simulink model "Relu_NoOutFB_4_4_1_HW_C6"  (R2012b)
settings: Solver=FixedStepDiscrete  SolverMode=SingleTasking  StartTime=0.0  StopTime=limSim  FixedStep=ts  RelTol=1e-3
undefined symbols (not defined in the file): alpha, delayMulx, delayMuly, delayROMSig, M2, M3, mu, ts
libraries: xbsIndex_r4 x1578, roblocks x1
(part 10 of 13)

== system Relu_NoOutFB_4_4_1_HW_C6/EN_MLP_BK_(1,4_NL,1_L)_HW_FPGA2/MLP_BK_(2,4_NL,1_L)_HW_FPGA/BK (2,4_NL,1_L)/Subsystem8/Subsystem2 ==
  Gx_1(n) : Inport
  x_1(n) : Inport  Port=2
  AddSub1 : xbsIndex_r4/AddSub  mode=Addition  use_carryin=off  use_carryout=off  en=off  latency=0  precision=User Defined  arith_type="Signed  (2's comp)"  n_bits=nb  bin_pt=bp  quantization=Truncate  overflow=Wrap  dbl_ovrd=off  use_behavioral_HDL=off  hw_selection=Fabric  pipelined=off  block_type=addsub
  AddSub2 : xbsIndex_r4/AddSub  mode=Addition  use_carryin=off  use_carryout=off  en=off  latency=0  precision=User Defined  arith_type="Signed  (2's comp)"  n_bits=nb  bin_pt=bp  quantization=Truncate  overflow=Wrap  dbl_ovrd=off  use_behavioral_HDL=off  hw_selection=Fabric  pipelined=off  block_type=addsub
  CMult : xbsIndex_r4/CMult  const=mu  gui_display_data_type=Fixed-point  const_n_bits=32  const_bin_pt=32  float_type=Single  exp_bits=8  fraction_bits=24  en=off  latency=0  precision=User Defined  arith_type="Signed  (2's comp)"  n_bits=nb  bin_pt=bp  quantization="Round  (unbiased: +/- Inf)"  overflow=Wrap  dbl_ovrd=off  use_behavioral_HDL=off  mem_type=Distributed RAM  pipeline=off  block_type=cmult
  CMult2 : xbsIndex_r4/CMult  const=alpha  gui_display_data_type=Fixed-point  const_n_bits=32  const_bin_pt=32  float_type=Single  exp_bits=8  fraction_bits=24  en=off  latency=0  precision=User Defined  arith_type="Signed  (2's comp)"  n_bits=nb  bin_pt=bp  quantization="Round  (unbiased: +/- Inf)"  overflow=Wrap  dbl_ovrd=off  use_behavioral_HDL=off  mem_type=Distributed RAM  pipeline=off  block_type=cmult
  Register : xbsIndex_r4/Register  init=real(M3(1,4))  rst=off  en=off  dbl_ovrd=off  block_type=register
  Register1 : xbsIndex_r4/Register  init=0  rst=off  en=off  dbl_ovrd=off  block_type=register
  w_ij(n)*Gy(n)2 : xbsIndex_r4/Mult  precision=User Defined  arith_type="Signed  (2's comp)"  n_bits=nb  bin_pt=bp  quantization="Round  (unbiased: +/- Inf)"  overflow=Saturate  en=off  latency=delayMulx  dbl_ovrd=off  use_behavioral_HDL=off  opt=Speed  use_embedded=on  optimum_pipeline=off  pipeline=on  use_rpm=on  placement_style=Triangular  block_type=mult
  Wx_13(n) : Outport
  wires:
  x_1(n)/1 -> w_ij(n)*Gy(n)2/2
  w_ij(n)*Gy(n)2/1 -> CMult/1
  CMult/1 -> AddSub2/2  "dw(n) = z_0(n)*e(n)*mu"
  AddSub2/1 -> AddSub1/2
  AddSub1/1 -> Register/1  "w_ij(n+1)"
  Register1/1 -> CMult2/1  "w_ij(n-1)"
  CMult2/1 -> AddSub2/1  "alpha*w_ij(n-1)"
  Register/1 -> AddSub1/1, Register1/1, Wx_13(n)/1  "w_ij(n)"
  Gx_1(n)/1 -> w_ij(n)*Gy(n)2/1

== system Relu_NoOutFB_4_4_1_HW_C6/EN_MLP_BK_(1,4_NL,1_L)_HW_FPGA2/MLP_BK_(2,4_NL,1_L)_HW_FPGA/BK (2,4_NL,1_L)/Subsystem8/Subsystem3 ==
  Gx_1(n) : Inport
  x_1(n) : Inport  Port=2
  AddSub1 : xbsIndex_r4/AddSub  mode=Addition  use_carryin=off  use_carryout=off  en=off  latency=0  precision=User Defined  arith_type="Signed  (2's comp)"  n_bits=nb  bin_pt=bp  quantization=Truncate  overflow=Wrap  dbl_ovrd=off  use_behavioral_HDL=off  hw_selection=Fabric  pipelined=off  block_type=addsub
  AddSub2 : xbsIndex_r4/AddSub  mode=Addition  use_carryin=off  use_carryout=off  en=off  latency=0  precision=User Defined  arith_type="Signed  (2's comp)"  n_bits=nb  bin_pt=bp  quantization=Truncate  overflow=Wrap  dbl_ovrd=off  use_behavioral_HDL=off  hw_selection=Fabric  pipelined=off  block_type=addsub
  CMult : xbsIndex_r4/CMult  const=mu  gui_display_data_type=Fixed-point  const_n_bits=32  const_bin_pt=32  float_type=Single  exp_bits=8  fraction_bits=24  en=off  latency=0  precision=User Defined  arith_type="Signed  (2's comp)"  n_bits=nb  bin_pt=bp  quantization="Round  (unbiased: +/- Inf)"  overflow=Wrap  dbl_ovrd=off  use_behavioral_HDL=off  mem_type=Distributed RAM  pipeline=off  block_type=cmult
  CMult2 : xbsIndex_r4/CMult  const=alpha  gui_display_data_type=Fixed-point  const_n_bits=32  const_bin_pt=32  float_type=Single  exp_bits=8  fraction_bits=24  en=off  latency=0  precision=User Defined  arith_type="Signed  (2's comp)"  n_bits=nb  bin_pt=bp  quantization="Round  (unbiased: +/- Inf)"  overflow=Wrap  dbl_ovrd=off  use_behavioral_HDL=off  mem_type=Distributed RAM  pipeline=off  block_type=cmult
  Register : xbsIndex_r4/Register  init=real(M3(1,5))  rst=off  en=off  dbl_ovrd=off  block_type=register
  Register1 : xbsIndex_r4/Register  init=0  rst=off  en=off  dbl_ovrd=off  block_type=register
  w_ij(n)*Gy(n)2 : xbsIndex_r4/Mult  precision=User Defined  arith_type="Signed  (2's comp)"  n_bits=nb  bin_pt=bp  quantization="Round  (unbiased: +/- Inf)"  overflow=Saturate  en=off  latency=delayMulx  dbl_ovrd=off  use_behavioral_HDL=off  opt=Speed  use_embedded=on  optimum_pipeline=off  pipeline=on  use_rpm=on  placement_style=Triangular  block_type=mult
  Wx_14(n) : Outport
  wires:
  Gx_1(n)/1 -> w_ij(n)*Gy(n)2/1
  Register/1 -> Wx_14(n)/1, Register1/1, AddSub1/1  "w_ij(n)"
  CMult2/1 -> AddSub2/1  "alpha*w_ij(n-1)"
  Register1/1 -> CMult2/1  "w_ij(n-1)"
  AddSub1/1 -> Register/1  "w_ij(n+1)"
  AddSub2/1 -> AddSub1/2
  CMult/1 -> AddSub2/2  "dw(n) = z_0(n)*e(n)*mu"
  w_ij(n)*Gy(n)2/1 -> CMult/1
  x_1(n)/1 -> w_ij(n)*Gy(n)2/2

== system Relu_NoOutFB_4_4_1_HW_C6/EN_MLP_BK_(1,4_NL,1_L)_HW_FPGA2/MLP_BK_(2,4_NL,1_L)_HW_FPGA/BK (2,4_NL,1_L)/Subsystem8/Subsystem5 ==
  Gx_1(n) : Inport
  x_0(n) : Inport  Port=2
  AddSub1 : xbsIndex_r4/AddSub  mode=Addition  use_carryin=off  use_carryout=off  en=off  latency=0  precision=User Defined  arith_type="Signed  (2's comp)"  n_bits=nb  bin_pt=bp  quantization=Truncate  overflow=Wrap  dbl_ovrd=off  use_behavioral_HDL=off  hw_selection=Fabric  pipelined=off  block_type=addsub
  AddSub2 : xbsIndex_r4/AddSub  mode=Addition  use_carryin=off  use_carryout=off  en=off  latency=0  precision=User Defined  arith_type="Signed  (2's comp)"  n_bits=nb  bin_pt=bp  quantization=Truncate  overflow=Wrap  dbl_ovrd=off  use_behavioral_HDL=off  hw_selection=Fabric  pipelined=off  block_type=addsub
  CMult : xbsIndex_r4/CMult  const=mu  gui_display_data_type=Fixed-point  const_n_bits=32  const_bin_pt=32  float_type=Single  exp_bits=8  fraction_bits=24  en=off  latency=0  precision=User Defined  arith_type="Signed  (2's comp)"  n_bits=nb  bin_pt=bp  quantization="Round  (unbiased: +/- Inf)"  overflow=Wrap  dbl_ovrd=off  use_behavioral_HDL=off  mem_type=Distributed RAM  pipeline=off  block_type=cmult
  CMult2 : xbsIndex_r4/CMult  const=alpha  gui_display_data_type=Fixed-point  const_n_bits=32  const_bin_pt=32  float_type=Single  exp_bits=8  fraction_bits=24  en=off  latency=0  precision=User Defined  arith_type="Signed  (2's comp)"  n_bits=nb  bin_pt=bp  quantization="Round  (unbiased: +/- Inf)"  overflow=Wrap  dbl_ovrd=off  use_behavioral_HDL=off  mem_type=Distributed RAM  pipeline=off  block_type=cmult
  Register : xbsIndex_r4/Register  init=real(M3(1,1))  rst=off  en=off  dbl_ovrd=off  block_type=register
  Register1 : xbsIndex_r4/Register  init=0  rst=off  en=off  dbl_ovrd=off  block_type=register
  w_ij(n)*Gy(n)2 : xbsIndex_r4/Mult  precision=User Defined  arith_type="Signed  (2's comp)"  n_bits=nb  bin_pt=bp  quantization="Round  (unbiased: +/- Inf)"  overflow=Saturate  en=off  latency=delayMulx  dbl_ovrd=off  use_behavioral_HDL=off  opt=Speed  use_embedded=on  optimum_pipeline=off  pipeline=on  use_rpm=on  placement_style=Triangular  block_type=mult
  Wx_10(n) : Outport
  wires:
  Gx_1(n)/1 -> w_ij(n)*Gy(n)2/1
  Register/1 -> Wx_10(n)/1, Register1/1, AddSub1/1  "w_ij(n)"
  CMult2/1 -> AddSub2/1  "alpha*w_ij(n-1)"
  Register1/1 -> CMult2/1  "w_ij(n-1)"
  AddSub1/1 -> Register/1  "w_ij(n+1)"
  AddSub2/1 -> AddSub1/2
  CMult/1 -> AddSub2/2  "dw(n) = z_0(n)*e(n)*mu"
  w_ij(n)*Gy(n)2/1 -> CMult/1
  x_0(n)/1 -> w_ij(n)*Gy(n)2/2

== system Relu_NoOutFB_4_4_1_HW_C6/EN_MLP_BK_(1,4_NL,1_L)_HW_FPGA2/MLP_BK_(2,4_NL,1_L)_HW_FPGA/BK (2,4_NL,1_L)/Subsystem8/Subsystem6 ==
  Gx_1(n) : Inport
  x_1(n) : Inport  Port=2
  AddSub1 : xbsIndex_r4/AddSub  mode=Addition  use_carryin=off  use_carryout=off  en=off  latency=0  precision=User Defined  arith_type="Signed  (2's comp)"  n_bits=nb  bin_pt=bp  quantization=Truncate  overflow=Wrap  dbl_ovrd=off  use_behavioral_HDL=off  hw_selection=Fabric  pipelined=off  block_type=addsub
  AddSub2 : xbsIndex_r4/AddSub  mode=Addition  use_carryin=off  use_carryout=off  en=off  latency=0  precision=User Defined  arith_type="Signed  (2's comp)"  n_bits=nb  bin_pt=bp  quantization=Truncate  overflow=Wrap  dbl_ovrd=off  use_behavioral_HDL=off  hw_selection=Fabric  pipelined=off  block_type=addsub
  CMult : xbsIndex_r4/CMult  const=mu  gui_display_data_type=Fixed-point  const_n_bits=32  const_bin_pt=32  float_type=Single  exp_bits=8  fraction_bits=24  en=off  latency=0  precision=User Defined  arith_type="Signed  (2's comp)"  n_bits=nb  bin_pt=bp  quantization="Round  (unbiased: +/- Inf)"  overflow=Wrap  dbl_ovrd=off  use_behavioral_HDL=off  mem_type=Distributed RAM  pipeline=off  block_type=cmult
  CMult2 : xbsIndex_r4/CMult  const=alpha  gui_display_data_type=Fixed-point  const_n_bits=32  const_bin_pt=32  float_type=Single  exp_bits=8  fraction_bits=24  en=off  latency=0  precision=User Defined  arith_type="Signed  (2's comp)"  n_bits=nb  bin_pt=bp  quantization="Round  (unbiased: +/- Inf)"  overflow=Wrap  dbl_ovrd=off  use_behavioral_HDL=off  mem_type=Distributed RAM  pipeline=off  block_type=cmult
  Register : xbsIndex_r4/Register  init=real(M3(1,2))  rst=off  en=off  dbl_ovrd=off  block_type=register
  Register1 : xbsIndex_r4/Register  init=0  rst=off  en=off  dbl_ovrd=off  block_type=register
  w_ij(n)*Gy(n)2 : xbsIndex_r4/Mult  precision=User Defined  arith_type="Signed  (2's comp)"  n_bits=nb  bin_pt=bp  quantization="Round  (unbiased: +/- Inf)"  overflow=Saturate  en=off  latency=delayMulx  dbl_ovrd=off  use_behavioral_HDL=off  opt=Speed  use_embedded=on  optimum_pipeline=off  pipeline=on  use_rpm=on  placement_style=Triangular  block_type=mult
  Wx_11(n) : Outport
  wires:
  x_1(n)/1 -> w_ij(n)*Gy(n)2/2
  w_ij(n)*Gy(n)2/1 -> CMult/1
  CMult/1 -> AddSub2/2  "dw(n) = z_0(n)*e(n)*mu"
  AddSub2/1 -> AddSub1/2
  AddSub1/1 -> Register/1  "w_ij(n+1)"
  Register1/1 -> CMult2/1  "w_ij(n-1)"
  CMult2/1 -> AddSub2/1  "alpha*w_ij(n-1)"
  Register/1 -> AddSub1/1, Register1/1, Wx_11(n)/1  "w_ij(n)"
  Gx_1(n)/1 -> w_ij(n)*Gy(n)2/1

== system Relu_NoOutFB_4_4_1_HW_C6/EN_MLP_BK_(1,4_NL,1_L)_HW_FPGA2/MLP_BK_(2,4_NL,1_L)_HW_FPGA/MLP (2,4_NL,1_L)/Neurônio Não-Linear_HW1/Subsystem ==
  In1 : Inport
  Constant : xbsIndex_r4/Constant  const=0  gui_display_data_type=Fixed-point  arith_type=Signed (2's comp)  n_bits=nb  bin_pt=bp  preci_type=Single  exp_width=8  frac_width=24  explicit_period=off  period=1  equ=P=C  opselect=C  inp2=PCIN>>17  opr=+  inp1=P  carry=CIN  dbl_ovrd=off  block_type=constant
  Mux : xbsIndex_r4/Mux  inputs=2  en=off  latency=0  precision=Full  arith_type=Unsigned  n_bits=16  bin_pt=14  quantization=Truncate  overflow=Wrap  dbl_ovrd=off  block_type=mux
  Relational : xbsIndex_r4/Relational  mode=a>b  en=off  latency=0  dbl_ovrd=off  block_type=relational
  Out1 : Outport
  wires:
  Constant/1 -> Mux/2, Relational/2
  Relational/1 -> Mux/1
  In1/1 -> Relational/1, Mux/3
  Mux/1 -> Out1/1

== system Relu_NoOutFB_4_4_1_HW_C6/EN_MLP_BK_(1,4_NL,1_L)_HW_FPGA2/MLP_BK_(2,4_NL,1_L)_HW_FPGA/MLP (2,4_NL,1_L)/Neurônio Não-Linear_HW2/Subsystem ==
  In1 : Inport
  Constant : xbsIndex_r4/Constant  const=0  gui_display_data_type=Fixed-point  arith_type=Signed (2's comp)  n_bits=nb  bin_pt=bp  preci_type=Single  exp_width=8  frac_width=24  explicit_period=off  period=1  equ=P=C  opselect=C  inp2=PCIN>>17  opr=+  inp1=P  carry=CIN  dbl_ovrd=off  block_type=constant
  Mux : xbsIndex_r4/Mux  inputs=2  en=off  latency=0  precision=Full  arith_type=Unsigned  n_bits=16  bin_pt=14  quantization=Truncate  overflow=Wrap  dbl_ovrd=off  block_type=mux
  Relational : xbsIndex_r4/Relational  mode=a>b  en=off  latency=0  dbl_ovrd=off  block_type=relational
  Out1 : Outport
  wires:
  Constant/1 -> Mux/2, Relational/2
  Relational/1 -> Mux/1
  In1/1 -> Relational/1, Mux/3
  Mux/1 -> Out1/1

== system Relu_NoOutFB_4_4_1_HW_C6/EN_MLP_BK_(1,4_NL,1_L)_HW_FPGA2/MLP_BK_(2,4_NL,1_L)_HW_FPGA/MLP (2,4_NL,1_L)/Neurônio Não-Linear_HW3/Subsystem ==
  In1 : Inport
  Constant : xbsIndex_r4/Constant  const=0  gui_display_data_type=Fixed-point  arith_type=Signed (2's comp)  n_bits=nb  bin_pt=bp  preci_type=Single  exp_width=8  frac_width=24  explicit_period=off  period=1  equ=P=C  opselect=C  inp2=PCIN>>17  opr=+  inp1=P  carry=CIN  dbl_ovrd=off  block_type=constant
  Mux : xbsIndex_r4/Mux  inputs=2  en=off  latency=0  precision=Full  arith_type=Unsigned  n_bits=16  bin_pt=14  quantization=Truncate  overflow=Wrap  dbl_ovrd=off  block_type=mux
  Relational : xbsIndex_r4/Relational  mode=a>b  en=off  latency=0  dbl_ovrd=off  block_type=relational
  Out1 : Outport
  wires:
  Constant/1 -> Mux/2, Relational/2
  Relational/1 -> Mux/1
  In1/1 -> Relational/1, Mux/3
  Mux/1 -> Out1/1

== system Relu_NoOutFB_4_4_1_HW_C6/EN_MLP_BK_(1,4_NL,1_L)_HW_FPGA2/MLP_BK_(2,4_NL,1_L)_HW_FPGA/MLP (2,4_NL,1_L)/Neurônio Não-Linear_HW4/Subsystem ==
  In1 : Inport
  Constant : xbsIndex_r4/Constant  const=0  gui_display_data_type=Fixed-point  arith_type=Signed (2's comp)  n_bits=nb  bin_pt=bp  preci_type=Single  exp_width=8  frac_width=24  explicit_period=off  period=1  equ=P=C  opselect=C  inp2=PCIN>>17  opr=+  inp1=P  carry=CIN  dbl_ovrd=off  block_type=constant
  Mux : xbsIndex_r4/Mux  inputs=2  en=off  latency=0  precision=Full  arith_type=Unsigned  n_bits=16  bin_pt=14  quantization=Truncate  overflow=Wrap  dbl_ovrd=off  block_type=mux
  Relational : xbsIndex_r4/Relational  mode=a>b  en=off  latency=0  dbl_ovrd=off  block_type=relational
  Out1 : Outport
  wires:
  Constant/1 -> Mux/2, Relational/2
  Relational/1 -> Mux/1
  In1/1 -> Relational/1, Mux/3
  Mux/1 -> Out1/1

== system Relu_NoOutFB_4_4_1_HW_C6/EN_MLP_BK_(1,4_NL,1_L)_HW_FPGA3/MLP_BK_(2,4_NL,1_L)_HW_FPGA/BK (2,4_NL,1_L)/Subsystem2/Subsystem1 ==
  Gx_1(n) : Inport
  x_1(n) : Inport  Port=2
  AddSub1 : xbsIndex_r4/AddSub  mode=Addition  use_carryin=off  use_carryout=off  en=off  latency=0  precision=User Defined  arith_type="Signed  (2's comp)"  n_bits=nb  bin_pt=bp  quantization=Truncate  overflow=Wrap  dbl_ovrd=off  use_behavioral_HDL=off  hw_selection=Fabric  pipelined=off  block_type=addsub
  AddSub2 : xbsIndex_r4/AddSub  mode=Addition  use_carryin=off  use_carryout=off  en=off  latency=0  precision=User Defined  arith_type="Signed  (2's comp)"  n_bits=nb  bin_pt=bp  quantization=Truncate  overflow=Wrap  dbl_ovrd=off  use_behavioral_HDL=off  hw_selection=Fabric  pipelined=off  block_type=addsub
  CMult : xbsIndex_r4/CMult  const=mu  gui_display_data_type=Fixed-point  const_n_bits=32  const_bin_pt=32  float_type=Single  exp_bits=8  fraction_bits=24  en=off  latency=0  precision=User Defined  arith_type="Signed  (2's comp)"  n_bits=nb  bin_pt=bp  quantization="Round  (unbiased: +/- Inf)"  overflow=Wrap  dbl_ovrd=off  use_behavioral_HDL=off  mem_type=Distributed RAM  pipeline=off  block_type=cmult
  CMult2 : xbsIndex_r4/CMult  const=alpha  gui_display_data_type=Fixed-point  const_n_bits=32  const_bin_pt=32  float_type=Single  exp_bits=8  fraction_bits=24  en=off  latency=0  precision=User Defined  arith_type="Signed  (2's comp)"  n_bits=nb  bin_pt=bp  quantization="Round  (unbiased: +/- Inf)"  overflow=Wrap  dbl_ovrd=off  use_behavioral_HDL=off  mem_type=Distributed RAM  pipeline=off  block_type=cmult
  Register : xbsIndex_r4/Register  init=real(M3(1,3))  rst=off  en=off  dbl_ovrd=off  block_type=register
  Register1 : xbsIndex_r4/Register  init=0  rst=off  en=off  dbl_ovrd=off  block_type=register
  w_ij(n)*Gy(n)2 : xbsIndex_r4/Mult  precision=User Defined  arith_type="Signed  (2's comp)"  n_bits=nb  bin_pt=bp  quantization="Round  (unbiased: +/- Inf)"  overflow=Saturate  en=off  latency=delayMulx  dbl_ovrd=off  use_behavioral_HDL=off  opt=Speed  use_embedded=on  optimum_pipeline=off  pipeline=on  use_rpm=on  placement_style=Triangular  block_type=mult
  Wx_11(n) : Outport
  wires:
  Gx_1(n)/1 -> w_ij(n)*Gy(n)2/1
  Register/1 -> Wx_11(n)/1, Register1/1, AddSub1/1  "w_ij(n)"
  CMult2/1 -> AddSub2/1  "alpha*w_ij(n-1)"
  Register1/1 -> CMult2/1  "w_ij(n-1)"
  AddSub1/1 -> Register/1  "w_ij(n+1)"
  AddSub2/1 -> AddSub1/2
  CMult/1 -> AddSub2/2  "dw(n) = z_0(n)*e(n)*mu"
  w_ij(n)*Gy(n)2/1 -> CMult/1
  x_1(n)/1 -> w_ij(n)*Gy(n)2/2

== system Relu_NoOutFB_4_4_1_HW_C6/EN_MLP_BK_(1,4_NL,1_L)_HW_FPGA3/MLP_BK_(2,4_NL,1_L)_HW_FPGA/BK (2,4_NL,1_L)/Subsystem2/Subsystem2 ==
  Gx_1(n) : Inport
  x_1(n) : Inport  Port=2
  AddSub1 : xbsIndex_r4/AddSub  mode=Addition  use_carryin=off  use_carryout=off  en=off  latency=0  precision=User Defined  arith_type="Signed  (2's comp)"  n_bits=nb  bin_pt=bp  quantization=Truncate  overflow=Wrap  dbl_ovrd=off  use_behavioral_HDL=off  hw_selection=Fabric  pipelined=off  block_type=addsub
  AddSub2 : xbsIndex_r4/AddSub  mode=Addition  use_carryin=off  use_carryout=off  en=off  latency=0  precision=User Defined  arith_type="Signed  (2's comp)"  n_bits=nb  bin_pt=bp  quantization=Truncate  overflow=Wrap  dbl_ovrd=off  use_behavioral_HDL=off  hw_selection=Fabric  pipelined=off  block_type=addsub
  CMult : xbsIndex_r4/CMult  const=mu  gui_display_data_type=Fixed-point  const_n_bits=32  const_bin_pt=32  float_type=Single  exp_bits=8  fraction_bits=24  en=off  latency=0  precision=User Defined  arith_type="Signed  (2's comp)"  n_bits=nb  bin_pt=bp  quantization="Round  (unbiased: +/- Inf)"  overflow=Wrap  dbl_ovrd=off  use_behavioral_HDL=off  mem_type=Distributed RAM  pipeline=off  block_type=cmult
  CMult2 : xbsIndex_r4/CMult  const=alpha  gui_display_data_type=Fixed-point  const_n_bits=32  const_bin_pt=32  float_type=Single  exp_bits=8  fraction_bits=24  en=off  latency=0  precision=User Defined  arith_type="Signed  (2's comp)"  n_bits=nb  bin_pt=bp  quantization="Round  (unbiased: +/- Inf)"  overflow=Wrap  dbl_ovrd=off  use_behavioral_HDL=off  mem_type=Distributed RAM  pipeline=off  block_type=cmult
  Register : xbsIndex_r4/Register  init=real(M3(1,4))  rst=off  en=off  dbl_ovrd=off  block_type=register
  Register1 : xbsIndex_r4/Register  init=0  rst=off  en=off  dbl_ovrd=off  block_type=register
  w_ij(n)*Gy(n)2 : xbsIndex_r4/Mult  precision=User Defined  arith_type="Signed  (2's comp)"  n_bits=nb  bin_pt=bp  quantization="Round  (unbiased: +/- Inf)"  overflow=Saturate  en=off  latency=delayMulx  dbl_ovrd=off  use_behavioral_HDL=off  opt=Speed  use_embedded=on  optimum_pipeline=off  pipeline=on  use_rpm=on  placement_style=Triangular  block_type=mult
  Wx_11(n) : Outport
  wires:
  x_1(n)/1 -> w_ij(n)*Gy(n)2/2
  w_ij(n)*Gy(n)2/1 -> CMult/1
  CMult/1 -> AddSub2/2  "dw(n) = z_0(n)*e(n)*mu"
  AddSub2/1 -> AddSub1/2
  AddSub1/1 -> Register/1  "w_ij(n+1)"
  Register1/1 -> CMult2/1  "w_ij(n-1)"
  CMult2/1 -> AddSub2/1  "alpha*w_ij(n-1)"
  Register/1 -> AddSub1/1, Register1/1, Wx_11(n)/1  "w_ij(n)"
  Gx_1(n)/1 -> w_ij(n)*Gy(n)2/1

== system Relu_NoOutFB_4_4_1_HW_C6/EN_MLP_BK_(1,4_NL,1_L)_HW_FPGA3/MLP_BK_(2,4_NL,1_L)_HW_FPGA/BK (2,4_NL,1_L)/Subsystem2/Subsystem3 ==
  Gx_1(n) : Inport
  x_1(n) : Inport  Port=2
  AddSub1 : xbsIndex_r4/AddSub  mode=Addition  use_carryin=off  use_carryout=off  en=off  latency=0  precision=User Defined  arith_type="Signed  (2's comp)"  n_bits=nb  bin_pt=bp  quantization=Truncate  overflow=Wrap  dbl_ovrd=off  use_behavioral_HDL=off  hw_selection=Fabric  pipelined=off  block_type=addsub
  AddSub2 : xbsIndex_r4/AddSub  mode=Addition  use_carryin=off  use_carryout=off  en=off  latency=0  precision=User Defined  arith_type="Signed  (2's comp)"  n_bits=nb  bin_pt=bp  quantization=Truncate  overflow=Wrap  dbl_ovrd=off  use_behavioral_HDL=off  hw_selection=Fabric  pipelined=off  block_type=addsub
  CMult : xbsIndex_r4/CMult  const=mu  gui_display_data_type=Fixed-point  const_n_bits=32  const_bin_pt=32  float_type=Single  exp_bits=8  fraction_bits=24  en=off  latency=0  precision=User Defined  arith_type="Signed  (2's comp)"  n_bits=nb  bin_pt=bp  quantization="Round  (unbiased: +/- Inf)"  overflow=Wrap  dbl_ovrd=off  use_behavioral_HDL=off  mem_type=Distributed RAM  pipeline=off  block_type=cmult
  CMult2 : xbsIndex_r4/CMult  const=alpha  gui_display_data_type=Fixed-point  const_n_bits=32  const_bin_pt=32  float_type=Single  exp_bits=8  fraction_bits=24  en=off  latency=0  precision=User Defined  arith_type="Signed  (2's comp)"  n_bits=nb  bin_pt=bp  quantization="Round  (unbiased: +/- Inf)"  overflow=Wrap  dbl_ovrd=off  use_behavioral_HDL=off  mem_type=Distributed RAM  pipeline=off  block_type=cmult
  Register : xbsIndex_r4/Register  init=real(M3(1,5))  rst=off  en=off  dbl_ovrd=off  block_type=register
  Register1 : xbsIndex_r4/Register  init=0  rst=off  en=off  dbl_ovrd=off  block_type=register
  w_ij(n)*Gy(n)2 : xbsIndex_r4/Mult  precision=User Defined  arith_type="Signed  (2's comp)"  n_bits=nb  bin_pt=bp  quantization="Round  (unbiased: +/- Inf)"  overflow=Saturate  en=off  latency=delayMulx  dbl_ovrd=off  use_behavioral_HDL=off  opt=Speed  use_embedded=on  optimum_pipeline=off  pipeline=on  use_rpm=on  placement_style=Triangular  block_type=mult
  Wx_11(n) : Outport
  wires:
  Gx_1(n)/1 -> w_ij(n)*Gy(n)2/1
  Register/1 -> Wx_11(n)/1, Register1/1, AddSub1/1  "w_ij(n)"
  CMult2/1 -> AddSub2/1  "alpha*w_ij(n-1)"
  Register1/1 -> CMult2/1  "w_ij(n-1)"
  AddSub1/1 -> Register/1  "w_ij(n+1)"
  AddSub2/1 -> AddSub1/2
  CMult/1 -> AddSub2/2  "dw(n) = z_0(n)*e(n)*mu"
  w_ij(n)*Gy(n)2/1 -> CMult/1
  x_1(n)/1 -> w_ij(n)*Gy(n)2/2

== system Relu_NoOutFB_4_4_1_HW_C6/EN_MLP_BK_(1,4_NL,1_L)_HW_FPGA3/MLP_BK_(2,4_NL,1_L)_HW_FPGA/BK (2,4_NL,1_L)/Subsystem2/Subsystem5 ==
  Gx_1(n) : Inport
  x_0(n) : Inport  Port=2
  AddSub1 : xbsIndex_r4/AddSub  mode=Addition  use_carryin=off  use_carryout=off  en=off  latency=0  precision=User Defined  arith_type="Signed  (2's comp)"  n_bits=nb  bin_pt=bp  quantization=Truncate  overflow=Wrap  dbl_ovrd=off  use_behavioral_HDL=off  hw_selection=Fabric  pipelined=off  block_type=addsub
  AddSub2 : xbsIndex_r4/AddSub  mode=Addition  use_carryin=off  use_carryout=off  en=off  latency=0  precision=User Defined  arith_type="Signed  (2's comp)"  n_bits=nb  bin_pt=bp  quantization=Truncate  overflow=Wrap  dbl_ovrd=off  use_behavioral_HDL=off  hw_selection=Fabric  pipelined=off  block_type=addsub
  CMult : xbsIndex_r4/CMult  const=mu  gui_display_data_type=Fixed-point  const_n_bits=32  const_bin_pt=32  float_type=Single  exp_bits=8  fraction_bits=24  en=off  latency=0  precision=User Defined  arith_type="Signed  (2's comp)"  n_bits=nb  bin_pt=bp  quantization="Round  (unbiased: +/- Inf)"  overflow=Wrap  dbl_ovrd=off  use_behavioral_HDL=off  mem_type=Distributed RAM  pipeline=off  block_type=cmult
  CMult2 : xbsIndex_r4/CMult  const=alpha  gui_display_data_type=Fixed-point  const_n_bits=32  const_bin_pt=32  float_type=Single  exp_bits=8  fraction_bits=24  en=off  latency=0  precision=User Defined  arith_type="Signed  (2's comp)"  n_bits=nb  bin_pt=bp  quantization="Round  (unbiased: +/- Inf)"  overflow=Wrap  dbl_ovrd=off  use_behavioral_HDL=off  mem_type=Distributed RAM  pipeline=off  block_type=cmult
  Register : xbsIndex_r4/Register  init=real(M3(1,1))  rst=off  en=off  dbl_ovrd=off  block_type=register
  Register1 : xbsIndex_r4/Register  init=0  rst=off  en=off  dbl_ovrd=off  block_type=register
  w_ij(n)*Gy(n)2 : xbsIndex_r4/Mult  precision=User Defined  arith_type="Signed  (2's comp)"  n_bits=nb  bin_pt=bp  quantization="Round  (unbiased: +/- Inf)"  overflow=Saturate  en=off  latency=delayMulx  dbl_ovrd=off  use_behavioral_HDL=off  opt=Speed  use_embedded=on  optimum_pipeline=off  pipeline=on  use_rpm=on  placement_style=Triangular  block_type=mult
  Wx_10(n) : Outport
  wires:
  Gx_1(n)/1 -> w_ij(n)*Gy(n)2/1
  Register/1 -> Wx_10(n)/1, Register1/1, AddSub1/1  "w_ij(n)"
  CMult2/1 -> AddSub2/1  "alpha*w_ij(n-1)"
  Register1/1 -> CMult2/1  "w_ij(n-1)"
  AddSub1/1 -> Register/1  "w_ij(n+1)"
  AddSub2/1 -> AddSub1/2
  CMult/1 -> AddSub2/2  "dw(n) = z_0(n)*e(n)*mu"
  w_ij(n)*Gy(n)2/1 -> CMult/1
  x_0(n)/1 -> w_ij(n)*Gy(n)2/2

== system Relu_NoOutFB_4_4_1_HW_C6/EN_MLP_BK_(1,4_NL,1_L)_HW_FPGA3/MLP_BK_(2,4_NL,1_L)_HW_FPGA/BK (2,4_NL,1_L)/Subsystem2/Subsystem6 ==
  Gx_1(n) : Inport
  x_1(n) : Inport  Port=2
  AddSub1 : xbsIndex_r4/AddSub  mode=Addition  use_carryin=off  use_carryout=off  en=off  latency=0  precision=User Defined  arith_type="Signed  (2's comp)"  n_bits=nb  bin_pt=bp  quantization=Truncate  overflow=Wrap  dbl_ovrd=off  use_behavioral_HDL=off  hw_selection=Fabric  pipelined=off  block_type=addsub
  AddSub2 : xbsIndex_r4/AddSub  mode=Addition  use_carryin=off  use_carryout=off  en=off  latency=0  precision=User Defined  arith_type="Signed  (2's comp)"  n_bits=nb  bin_pt=bp  quantization=Truncate  overflow=Wrap  dbl_ovrd=off  use_behavioral_HDL=off  hw_selection=Fabric  pipelined=off  block_type=addsub
  CMult : xbsIndex_r4/CMult  const=mu  gui_display_data_type=Fixed-point  const_n_bits=32  const_bin_pt=32  float_type=Single  exp_bits=8  fraction_bits=24  en=off  latency=0  precision=User Defined  arith_type="Signed  (2's comp)"  n_bits=nb  bin_pt=bp  quantization="Round  (unbiased: +/- Inf)"  overflow=Wrap  dbl_ovrd=off  use_behavioral_HDL=off  mem_type=Distributed RAM  pipeline=off  block_type=cmult
  CMult2 : xbsIndex_r4/CMult  const=alpha  gui_display_data_type=Fixed-point  const_n_bits=32  const_bin_pt=32  float_type=Single  exp_bits=8  fraction_bits=24  en=off  latency=0  precision=User Defined  arith_type="Signed  (2's comp)"  n_bits=nb  bin_pt=bp  quantization="Round  (unbiased: +/- Inf)"  overflow=Wrap  dbl_ovrd=off  use_behavioral_HDL=off  mem_type=Distributed RAM  pipeline=off  block_type=cmult
  Register : xbsIndex_r4/Register  init=real(M3(1,2))  rst=off  en=off  dbl_ovrd=off  block_type=register
  Register1 : xbsIndex_r4/Register  init=0  rst=off  en=off  dbl_ovrd=off  block_type=register
  w_ij(n)*Gy(n)2 : xbsIndex_r4/Mult  precision=User Defined  arith_type="Signed  (2's comp)"  n_bits=nb  bin_pt=bp  quantization="Round  (unbiased: +/- Inf)"  overflow=Saturate  en=off  latency=delayMulx  dbl_ovrd=off  use_behavioral_HDL=off  opt=Speed  use_embedded=on  optimum_pipeline=off  pipeline=on  use_rpm=on  placement_style=Triangular  block_type=mult
  Wx_11(n) : Outport
  wires:
  x_1(n)/1 -> w_ij(n)*Gy(n)2/2
  w_ij(n)*Gy(n)2/1 -> CMult/1
  CMult/1 -> AddSub2/2  "dw(n) = z_0(n)*e(n)*mu"
  AddSub2/1 -> AddSub1/2
  AddSub1/1 -> Register/1  "w_ij(n+1)"
  Register1/1 -> CMult2/1  "w_ij(n-1)"
  CMult2/1 -> AddSub2/1  "alpha*w_ij(n-1)"
  Register/1 -> AddSub1/1, Register1/1, Wx_11(n)/1  "w_ij(n)"
  Gx_1(n)/1 -> w_ij(n)*Gy(n)2/1

== system Relu_NoOutFB_4_4_1_HW_C6/EN_MLP_BK_(1,4_NL,1_L)_HW_FPGA3/MLP_BK_(2,4_NL,1_L)_HW_FPGA/BK (2,4_NL,1_L)/Subsystem5/Subsystem1 ==
  Gx_1(n) : Inport
  x_1(n) : Inport  Port=2
  AddSub1 : xbsIndex_r4/AddSub  mode=Addition  use_carryin=off  use_carryout=off  en=off  latency=0  precision=User Defined  arith_type="Signed  (2's comp)"  n_bits=nb  bin_pt=bp  quantization=Truncate  overflow=Wrap  dbl_ovrd=off  use_behavioral_HDL=off  hw_selection=Fabric  pipelined=off  block_type=addsub
  AddSub2 : xbsIndex_r4/AddSub  mode=Addition  use_carryin=off  use_carryout=off  en=off  latency=0  precision=User Defined  arith_type="Signed  (2's comp)"  n_bits=nb  bin_pt=bp  quantization=Truncate  overflow=Wrap  dbl_ovrd=off  use_behavioral_HDL=off  hw_selection=Fabric  pipelined=off  block_type=addsub
  CMult : xbsIndex_r4/CMult  const=mu  gui_display_data_type=Fixed-point  const_n_bits=32  const_bin_pt=32  float_type=Single  exp_bits=8  fraction_bits=24  en=off  latency=0  precision=User Defined  arith_type="Signed  (2's comp)"  n_bits=nb  bin_pt=bp  quantization="Round  (unbiased: +/- Inf)"  overflow=Wrap  dbl_ovrd=off  use_behavioral_HDL=off  mem_type=Distributed RAM  pipeline=off  block_type=cmult
  CMult2 : xbsIndex_r4/CMult  const=alpha  gui_display_data_type=Fixed-point  const_n_bits=32  const_bin_pt=32  float_type=Single  exp_bits=8  fraction_bits=24  en=off  latency=0  precision=User Defined  arith_type="Signed  (2's comp)"  n_bits=nb  bin_pt=bp  quantization="Round  (unbiased: +/- Inf)"  overflow=Wrap  dbl_ovrd=off  use_behavioral_HDL=off  mem_type=Distributed RAM  pipeline=off  block_type=cmult
  Register : xbsIndex_r4/Register  init=real(M3(1,3))  rst=off  en=off  dbl_ovrd=off  block_type=register
  Register1 : xbsIndex_r4/Register  init=0  rst=off  en=off  dbl_ovrd=off  block_type=register
  w_ij(n)*Gy(n)2 : xbsIndex_r4/Mult  precision=User Defined  arith_type="Signed  (2's comp)"  n_bits=nb  bin_pt=bp  quantization="Round  (unbiased: +/- Inf)"  overflow=Saturate  en=off  latency=delayMulx  dbl_ovrd=off  use_behavioral_HDL=off  opt=Speed  use_embedded=on  optimum_pipeline=off  pipeline=on  use_rpm=on  placement_style=Triangular  block_type=mult
  Wx_11(n) : Outport
  wires:
  x_1(n)/1 -> w_ij(n)*Gy(n)2/2
  w_ij(n)*Gy(n)2/1 -> CMult/1
  CMult/1 -> AddSub2/2  "dw(n) = z_0(n)*e(n)*mu"
  AddSub2/1 -> AddSub1/2
  AddSub1/1 -> Register/1  "w_ij(n+1)"
  Register1/1 -> CMult2/1  "w_ij(n-1)"
  CMult2/1 -> AddSub2/1  "alpha*w_ij(n-1)"
  Register/1 -> AddSub1/1, Register1/1, Wx_11(n)/1  "w_ij(n)"
  Gx_1(n)/1 -> w_ij(n)*Gy(n)2/1

== system Relu_NoOutFB_4_4_1_HW_C6/EN_MLP_BK_(1,4_NL,1_L)_HW_FPGA3/MLP_BK_(2,4_NL,1_L)_HW_FPGA/BK (2,4_NL,1_L)/Subsystem5/Subsystem2 ==
  Gx_1(n) : Inport
  x_1(n) : Inport  Port=2
  AddSub1 : xbsIndex_r4/AddSub  mode=Addition  use_carryin=off  use_carryout=off  en=off  latency=0  precision=User Defined  arith_type="Signed  (2's comp)"  n_bits=nb  bin_pt=bp  quantization=Truncate  overflow=Wrap  dbl_ovrd=off  use_behavioral_HDL=off  hw_selection=Fabric  pipelined=off  block_type=addsub
  AddSub2 : xbsIndex_r4/AddSub  mode=Addition  use_carryin=off  use_carryout=off  en=off  latency=0  precision=User Defined  arith_type="Signed  (2's comp)"  n_bits=nb  bin_pt=bp  quantization=Truncate  overflow=Wrap  dbl_ovrd=off  use_behavioral_HDL=off  hw_selection=Fabric  pipelined=off  block_type=addsub
  CMult : xbsIndex_r4/CMult  const=mu  gui_display_data_type=Fixed-point  const_n_bits=32  const_bin_pt=32  float_type=Single  exp_bits=8  fraction_bits=24  en=off  latency=0  precision=User Defined  arith_type="Signed  (2's comp)"  n_bits=nb  bin_pt=bp  quantization="Round  (unbiased: +/- Inf)"  overflow=Wrap  dbl_ovrd=off  use_behavioral_HDL=off  mem_type=Distributed RAM  pipeline=off  block_type=cmult
  CMult2 : xbsIndex_r4/CMult  const=alpha  gui_display_data_type=Fixed-point  const_n_bits=32  const_bin_pt=32  float_type=Single  exp_bits=8  fraction_bits=24  en=off  latency=0  precision=User Defined  arith_type="Signed  (2's comp)"  n_bits=nb  bin_pt=bp  quantization="Round  (unbiased: +/- Inf)"  overflow=Wrap  dbl_ovrd=off  use_behavioral_HDL=off  mem_type=Distributed RAM  pipeline=off  block_type=cmult
  Register : xbsIndex_r4/Register  init=real(M3(1,4))  rst=off  en=off  dbl_ovrd=off  block_type=register
  Register1 : xbsIndex_r4/Register  init=0  rst=off  en=off  dbl_ovrd=off  block_type=register
  w_ij(n)*Gy(n)2 : xbsIndex_r4/Mult  precision=User Defined  arith_type="Signed  (2's comp)"  n_bits=nb  bin_pt=bp  quantization="Round  (unbiased: +/- Inf)"  overflow=Saturate  en=off  latency=delayMulx  dbl_ovrd=off  use_behavioral_HDL=off  opt=Speed  use_embedded=on  optimum_pipeline=off  pipeline=on  use_rpm=on  placement_style=Triangular  block_type=mult
  Wx_11(n) : Outport
  wires:
  Gx_1(n)/1 -> w_ij(n)*Gy(n)2/1
  Register/1 -> Wx_11(n)/1, Register1/1, AddSub1/1  "w_ij(n)"
  CMult2/1 -> AddSub2/1  "alpha*w_ij(n-1)"
  Register1/1 -> CMult2/1  "w_ij(n-1)"
  AddSub1/1 -> Register/1  "w_ij(n+1)"
  AddSub2/1 -> AddSub1/2
  CMult/1 -> AddSub2/2  "dw(n) = z_0(n)*e(n)*mu"
  w_ij(n)*Gy(n)2/1 -> CMult/1
  x_1(n)/1 -> w_ij(n)*Gy(n)2/2

== system Relu_NoOutFB_4_4_1_HW_C6/EN_MLP_BK_(1,4_NL,1_L)_HW_FPGA3/MLP_BK_(2,4_NL,1_L)_HW_FPGA/BK (2,4_NL,1_L)/Subsystem5/Subsystem3 ==
  Gx_1(n) : Inport
  x_1(n) : Inport  Port=2
  AddSub1 : xbsIndex_r4/AddSub  mode=Addition  use_carryin=off  use_carryout=off  en=off  latency=0  precision=User Defined  arith_type="Signed  (2's comp)"  n_bits=nb  bin_pt=bp  quantization=Truncate  overflow=Wrap  dbl_ovrd=off  use_behavioral_HDL=off  hw_selection=Fabric  pipelined=off  block_type=addsub
  AddSub2 : xbsIndex_r4/AddSub  mode=Addition  use_carryin=off  use_carryout=off  en=off  latency=0  precision=User Defined  arith_type="Signed  (2's comp)"  n_bits=nb  bin_pt=bp  quantization=Truncate  overflow=Wrap  dbl_ovrd=off  use_behavioral_HDL=off  hw_selection=Fabric  pipelined=off  block_type=addsub
  CMult : xbsIndex_r4/CMult  const=mu  gui_display_data_type=Fixed-point  const_n_bits=32  const_bin_pt=32  float_type=Single  exp_bits=8  fraction_bits=24  en=off  latency=0  precision=User Defined  arith_type="Signed  (2's comp)"  n_bits=nb  bin_pt=bp  quantization="Round  (unbiased: +/- Inf)"  overflow=Wrap  dbl_ovrd=off  use_behavioral_HDL=off  mem_type=Distributed RAM  pipeline=off  block_type=cmult
  CMult2 : xbsIndex_r4/CMult  const=alpha  gui_display_data_type=Fixed-point  const_n_bits=32  const_bin_pt=32  float_type=Single  exp_bits=8  fraction_bits=24  en=off  latency=0  precision=User Defined  arith_type="Signed  (2's comp)"  n_bits=nb  bin_pt=bp  quantization="Round  (unbiased: +/- Inf)"  overflow=Wrap  dbl_ovrd=off  use_behavioral_HDL=off  mem_type=Distributed RAM  pipeline=off  block_type=cmult
  Register : xbsIndex_r4/Register  init=real(M3(1,5))  rst=off  en=off  dbl_ovrd=off  block_type=register
  Register1 : xbsIndex_r4/Register  init=0  rst=off  en=off  dbl_ovrd=off  block_type=register
  w_ij(n)*Gy(n)2 : xbsIndex_r4/Mult  precision=User Defined  arith_type="Signed  (2's comp)"  n_bits=nb  bin_pt=bp  quantization="Round  (unbiased: +/- Inf)"  overflow=Saturate  en=off  latency=delayMulx  dbl_ovrd=off  use_behavioral_HDL=off  opt=Speed  use_embedded=on  optimum_pipeline=off  pipeline=on  use_rpm=on  placement_style=Triangular  block_type=mult
  Wx_11(n) : Outport
  wires:
  x_1(n)/1 -> w_ij(n)*Gy(n)2/2
  w_ij(n)*Gy(n)2/1 -> CMult/1
  CMult/1 -> AddSub2/2  "dw(n) = z_0(n)*e(n)*mu"
  AddSub2/1 -> AddSub1/2
  AddSub1/1 -> Register/1  "w_ij(n+1)"
  Register1/1 -> CMult2/1  "w_ij(n-1)"
  CMult2/1 -> AddSub2/1  "alpha*w_ij(n-1)"
  Register/1 -> AddSub1/1, Register1/1, Wx_11(n)/1  "w_ij(n)"
  Gx_1(n)/1 -> w_ij(n)*Gy(n)2/1

== system Relu_NoOutFB_4_4_1_HW_C6/EN_MLP_BK_(1,4_NL,1_L)_HW_FPGA3/MLP_BK_(2,4_NL,1_L)_HW_FPGA/BK (2,4_NL,1_L)/Subsystem5/Subsystem5 ==
  Gx_1(n) : Inport
  x_0(n) : Inport  Port=2
  AddSub1 : xbsIndex_r4/AddSub  mode=Addition  use_carryin=off  use_carryout=off  en=off  latency=0  precision=User Defined  arith_type="Signed  (2's comp)"  n_bits=nb  bin_pt=bp  quantization=Truncate  overflow=Wrap  dbl_ovrd=off  use_behavioral_HDL=off  hw_selection=Fabric  pipelined=off  block_type=addsub
  AddSub2 : xbsIndex_r4/AddSub  mode=Addition  use_carryin=off  use_carryout=off  en=off  latency=0  precision=User Defined  arith_type="Signed  (2's comp)"  n_bits=nb  bin_pt=bp  quantization=Truncate  overflow=Wrap  dbl_ovrd=off  use_behavioral_HDL=off  hw_selection=Fabric  pipelined=off  block_type=addsub
  CMult : xbsIndex_r4/CMult  const=mu  gui_display_data_type=Fixed-point  const_n_bits=32  const_bin_pt=32  float_type=Single  exp_bits=8  fraction_bits=24  en=off  latency=0  precision=User Defined  arith_type="Signed  (2's comp)"  n_bits=nb  bin_pt=bp  quantization="Round  (unbiased: +/- Inf)"  overflow=Wrap  dbl_ovrd=off  use_behavioral_HDL=off  mem_type=Distributed RAM  pipeline=off  block_type=cmult
  CMult2 : xbsIndex_r4/CMult  const=alpha  gui_display_data_type=Fixed-point  const_n_bits=32  const_bin_pt=32  float_type=Single  exp_bits=8  fraction_bits=24  en=off  latency=0  precision=User Defined  arith_type="Signed  (2's comp)"  n_bits=nb  bin_pt=bp  quantization="Round  (unbiased: +/- Inf)"  overflow=Wrap  dbl_ovrd=off  use_behavioral_HDL=off  mem_type=Distributed RAM  pipeline=off  block_type=cmult
  Register : xbsIndex_r4/Register  init=real(M3(1,1))  rst=off  en=off  dbl_ovrd=off  block_type=register
  Register1 : xbsIndex_r4/Register  init=0  rst=off  en=off  dbl_ovrd=off  block_type=register
  w_ij(n)*Gy(n)2 : xbsIndex_r4/Mult  precision=User Defined  arith_type="Signed  (2's comp)"  n_bits=nb  bin_pt=bp  quantization="Round  (unbiased: +/- Inf)"  overflow=Saturate  en=off  latency=delayMulx  dbl_ovrd=off  use_behavioral_HDL=off  opt=Speed  use_embedded=on  optimum_pipeline=off  pipeline=on  use_rpm=on  placement_style=Triangular  block_type=mult
  Wx_10(n) : Outport
  wires:
  x_0(n)/1 -> w_ij(n)*Gy(n)2/2
  w_ij(n)*Gy(n)2/1 -> CMult/1
  CMult/1 -> AddSub2/2  "dw(n) = z_0(n)*e(n)*mu"
  AddSub2/1 -> AddSub1/2
  AddSub1/1 -> Register/1  "w_ij(n+1)"
  Register1/1 -> CMult2/1  "w_ij(n-1)"
  CMult2/1 -> AddSub2/1  "alpha*w_ij(n-1)"
  Register/1 -> AddSub1/1, Register1/1, Wx_10(n)/1  "w_ij(n)"
  Gx_1(n)/1 -> w_ij(n)*Gy(n)2/1

== system Relu_NoOutFB_4_4_1_HW_C6/EN_MLP_BK_(1,4_NL,1_L)_HW_FPGA3/MLP_BK_(2,4_NL,1_L)_HW_FPGA/BK (2,4_NL,1_L)/Subsystem5/Subsystem6 ==
  Gx_1(n) : Inport
  x_1(n) : Inport  Port=2
  AddSub1 : xbsIndex_r4/AddSub  mode=Addition  use_carryin=off  use_carryout=off  en=off  latency=0  precision=User Defined  arith_type="Signed  (2's comp)"  n_bits=nb  bin_pt=bp  quantization=Truncate  overflow=Wrap  dbl_ovrd=off  use_behavioral_HDL=off  hw_selection=Fabric  pipelined=off  block_type=addsub
  AddSub2 : xbsIndex_r4/AddSub  mode=Addition  use_carryin=off  use_carryout=off  en=off  latency=0  precision=User Defined  arith_type="Signed  (2's comp)"  n_bits=nb  bin_pt=bp  quantization=Truncate  overflow=Wrap  dbl_ovrd=off  use_behavioral_HDL=off  hw_selection=Fabric  pipelined=off  block_type=addsub
  CMult : xbsIndex_r4/CMult  const=mu  gui_display_data_type=Fixed-point  const_n_bits=32  const_bin_pt=32  float_type=Single  exp_bits=8  fraction_bits=24  en=off  latency=0  precision=User Defined  arith_type="Signed  (2's comp)"  n_bits=nb  bin_pt=bp  quantization="Round  (unbiased: +/- Inf)"  overflow=Wrap  dbl_ovrd=off  use_behavioral_HDL=off  mem_type=Distributed RAM  pipeline=off  block_type=cmult
  CMult2 : xbsIndex_r4/CMult  const=alpha  gui_display_data_type=Fixed-point  const_n_bits=32  const_bin_pt=32  float_type=Single  exp_bits=8  fraction_bits=24  en=off  latency=0  precision=User Defined  arith_type="Signed  (2's comp)"  n_bits=nb  bin_pt=bp  quantization="Round  (unbiased: +/- Inf)"  overflow=Wrap  dbl_ovrd=off  use_behavioral_HDL=off  mem_type=Distributed RAM  pipeline=off  block_type=cmult
  Register : xbsIndex_r4/Register  init=real(M3(1,2))  rst=off  en=off  dbl_ovrd=off  block_type=register
  Register1 : xbsIndex_r4/Register  init=0  rst=off  en=off  dbl_ovrd=off  block_type=register
  w_ij(n)*Gy(n)2 : xbsIndex_r4/Mult  precision=User Defined  arith_type="Signed  (2's comp)"  n_bits=nb  bin_pt=bp  quantization="Round  (unbiased: +/- Inf)"  overflow=Saturate  en=off  latency=delayMulx  dbl_ovrd=off  use_behavioral_HDL=off  opt=Speed  use_embedded=on  optimum_pipeline=off  pipeline=on  use_rpm=on  placement_style=Triangular  block_type=mult
  Wx_11(n) : Outport
  wires:
  Gx_1(n)/1 -> w_ij(n)*Gy(n)2/1
  Register/1 -> Wx_11(n)/1, Register1/1, AddSub1/1  "w_ij(n)"
  CMult2/1 -> AddSub2/1  "alpha*w_ij(n-1)"
  Register1/1 -> CMult2/1  "w_ij(n-1)"
  AddSub1/1 -> Register/1  "w_ij(n+1)"
  AddSub2/1 -> AddSub1/2
  CMult/1 -> AddSub2/2  "dw(n) = z_0(n)*e(n)*mu"
  w_ij(n)*Gy(n)2/1 -> CMult/1
  x_1(n)/1 -> w_ij(n)*Gy(n)2/2

== system Relu_NoOutFB_4_4_1_HW_C6/EN_MLP_BK_(1,4_NL,1_L)_HW_FPGA3/MLP_BK_(2,4_NL,1_L)_HW_FPGA/BK (2,4_NL,1_L)/Subsystem6/Subsystem1 ==
  Gx_1(n) : Inport
  x_1(n) : Inport  Port=2
  AddSub1 : xbsIndex_r4/AddSub  mode=Addition  use_carryin=off  use_carryout=off  en=off  latency=0  precision=User Defined  arith_type="Signed  (2's comp)"  n_bits=nb  bin_pt=bp  quantization=Truncate  overflow=Wrap  dbl_ovrd=off  use_behavioral_HDL=off  hw_selection=Fabric  pipelined=off  block_type=addsub
  AddSub2 : xbsIndex_r4/AddSub  mode=Addition  use_carryin=off  use_carryout=off  en=off  latency=0  precision=User Defined  arith_type="Signed  (2's comp)"  n_bits=nb  bin_pt=bp  quantization=Truncate  overflow=Wrap  dbl_ovrd=off  use_behavioral_HDL=off  hw_selection=Fabric  pipelined=off  block_type=addsub
  CMult : xbsIndex_r4/CMult  const=mu  gui_display_data_type=Fixed-point  const_n_bits=32  const_bin_pt=32  float_type=Single  exp_bits=8  fraction_bits=24  en=off  latency=0  precision=User Defined  arith_type="Signed  (2's comp)"  n_bits=nb  bin_pt=bp  quantization="Round  (unbiased: +/- Inf)"  overflow=Wrap  dbl_ovrd=off  use_behavioral_HDL=off  mem_type=Distributed RAM  pipeline=off  block_type=cmult
  CMult2 : xbsIndex_r4/CMult  const=alpha  gui_display_data_type=Fixed-point  const_n_bits=32  const_bin_pt=32  float_type=Single  exp_bits=8  fraction_bits=24  en=off  latency=0  precision=User Defined  arith_type="Signed  (2's comp)"  n_bits=nb  bin_pt=bp  quantization="Round  (unbiased: +/- Inf)"  overflow=Wrap  dbl_ovrd=off  use_behavioral_HDL=off  mem_type=Distributed RAM  pipeline=off  block_type=cmult
  Register : xbsIndex_r4/Register  init=real(M3(1,3))  rst=off  en=off  dbl_ovrd=off  block_type=register
  Register1 : xbsIndex_r4/Register  init=0  rst=off  en=off  dbl_ovrd=off  block_type=register
  w_ij(n)*Gy(n)2 : xbsIndex_r4/Mult  precision=User Defined  arith_type="Signed  (2's comp)"  n_bits=nb  bin_pt=bp  quantization="Round  (unbiased: +/- Inf)"  overflow=Saturate  en=off  latency=delayMulx  dbl_ovrd=off  use_behavioral_HDL=off  opt=Speed  use_embedded=on  optimum_pipeline=off  pipeline=on  use_rpm=on  placement_style=Triangular  block_type=mult
  Wx_11(n) : Outport
  wires:
  Gx_1(n)/1 -> w_ij(n)*Gy(n)2/1
  Register/1 -> Wx_11(n)/1, Register1/1, AddSub1/1  "w_ij(n)"
  CMult2/1 -> AddSub2/1  "alpha*w_ij(n-1)"
  Register1/1 -> CMult2/1  "w_ij(n-1)"
  AddSub1/1 -> Register/1  "w_ij(n+1)"
  AddSub2/1 -> AddSub1/2
  CMult/1 -> AddSub2/2  "dw(n) = z_0(n)*e(n)*mu"
  w_ij(n)*Gy(n)2/1 -> CMult/1
  x_1(n)/1 -> w_ij(n)*Gy(n)2/2

== system Relu_NoOutFB_4_4_1_HW_C6/EN_MLP_BK_(1,4_NL,1_L)_HW_FPGA3/MLP_BK_(2,4_NL,1_L)_HW_FPGA/BK (2,4_NL,1_L)/Subsystem6/Subsystem2 ==
  Gx_1(n) : Inport
  x_1(n) : Inport  Port=2
  AddSub1 : xbsIndex_r4/AddSub  mode=Addition  use_carryin=off  use_carryout=off  en=off  latency=0  precision=User Defined  arith_type="Signed  (2's comp)"  n_bits=nb  bin_pt=bp  quantization=Truncate  overflow=Wrap  dbl_ovrd=off  use_behavioral_HDL=off  hw_selection=Fabric  pipelined=off  block_type=addsub
  AddSub2 : xbsIndex_r4/AddSub  mode=Addition  use_carryin=off  use_carryout=off  en=off  latency=0  precision=User Defined  arith_type="Signed  (2's comp)"  n_bits=nb  bin_pt=bp  quantization=Truncate  overflow=Wrap  dbl_ovrd=off  use_behavioral_HDL=off  hw_selection=Fabric  pipelined=off  block_type=addsub
  CMult : xbsIndex_r4/CMult  const=mu  gui_display_data_type=Fixed-point  const_n_bits=32  const_bin_pt=32  float_type=Single  exp_bits=8  fraction_bits=24  en=off  latency=0  precision=User Defined  arith_type="Signed  (2's comp)"  n_bits=nb  bin_pt=bp  quantization="Round  (unbiased: +/- Inf)"  overflow=Wrap  dbl_ovrd=off  use_behavioral_HDL=off  mem_type=Distributed RAM  pipeline=off  block_type=cmult
  CMult2 : xbsIndex_r4/CMult  const=alpha  gui_display_data_type=Fixed-point  const_n_bits=32  const_bin_pt=32  float_type=Single  exp_bits=8  fraction_bits=24  en=off  latency=0  precision=User Defined  arith_type="Signed  (2's comp)"  n_bits=nb  bin_pt=bp  quantization="Round  (unbiased: +/- Inf)"  overflow=Wrap  dbl_ovrd=off  use_behavioral_HDL=off  mem_type=Distributed RAM  pipeline=off  block_type=cmult
  Register : xbsIndex_r4/Register  init=real(M3(1,4))  rst=off  en=off  dbl_ovrd=off  block_type=register
  Register1 : xbsIndex_r4/Register  init=0  rst=off  en=off  dbl_ovrd=off  block_type=register
  w_ij(n)*Gy(n)2 : xbsIndex_r4/Mult  precision=User Defined  arith_type="Signed  (2's comp)"  n_bits=nb  bin_pt=bp  quantization="Round  (unbiased: +/- Inf)"  overflow=Saturate  en=off  latency=delayMulx  dbl_ovrd=off  use_behavioral_HDL=off  opt=Speed  use_embedded=on  optimum_pipeline=off  pipeline=on  use_rpm=on  placement_style=Triangular  block_type=mult
  Wx_11(n) : Outport
  wires:
  x_1(n)/1 -> w_ij(n)*Gy(n)2/2
  w_ij(n)*Gy(n)2/1 -> CMult/1
  CMult/1 -> AddSub2/2  "dw(n) = z_0(n)*e(n)*mu"
  AddSub2/1 -> AddSub1/2
  AddSub1/1 -> Register/1  "w_ij(n+1)"
  Register1/1 -> CMult2/1  "w_ij(n-1)"
  CMult2/1 -> AddSub2/1  "alpha*w_ij(n-1)"
  Register/1 -> AddSub1/1, Register1/1, Wx_11(n)/1  "w_ij(n)"
  Gx_1(n)/1 -> w_ij(n)*Gy(n)2/1

== system Relu_NoOutFB_4_4_1_HW_C6/EN_MLP_BK_(1,4_NL,1_L)_HW_FPGA3/MLP_BK_(2,4_NL,1_L)_HW_FPGA/BK (2,4_NL,1_L)/Subsystem6/Subsystem3 ==
  Gx_1(n) : Inport
  x_1(n) : Inport  Port=2
  AddSub1 : xbsIndex_r4/AddSub  mode=Addition  use_carryin=off  use_carryout=off  en=off  latency=0  precision=User Defined  arith_type="Signed  (2's comp)"  n_bits=nb  bin_pt=bp  quantization=Truncate  overflow=Wrap  dbl_ovrd=off  use_behavioral_HDL=off  hw_selection=Fabric  pipelined=off  block_type=addsub
  AddSub2 : xbsIndex_r4/AddSub  mode=Addition  use_carryin=off  use_carryout=off  en=off  latency=0  precision=User Defined  arith_type="Signed  (2's comp)"  n_bits=nb  bin_pt=bp  quantization=Truncate  overflow=Wrap  dbl_ovrd=off  use_behavioral_HDL=off  hw_selection=Fabric  pipelined=off  block_type=addsub
  CMult : xbsIndex_r4/CMult  const=mu  gui_display_data_type=Fixed-point  const_n_bits=32  const_bin_pt=32  float_type=Single  exp_bits=8  fraction_bits=24  en=off  latency=0  precision=User Defined  arith_type="Signed  (2's comp)"  n_bits=nb  bin_pt=bp  quantization="Round  (unbiased: +/- Inf)"  overflow=Wrap  dbl_ovrd=off  use_behavioral_HDL=off  mem_type=Distributed RAM  pipeline=off  block_type=cmult
  CMult2 : xbsIndex_r4/CMult  const=alpha  gui_display_data_type=Fixed-point  const_n_bits=32  const_bin_pt=32  float_type=Single  exp_bits=8  fraction_bits=24  en=off  latency=0  precision=User Defined  arith_type="Signed  (2's comp)"  n_bits=nb  bin_pt=bp  quantization="Round  (unbiased: +/- Inf)"  overflow=Wrap  dbl_ovrd=off  use_behavioral_HDL=off  mem_type=Distributed RAM  pipeline=off  block_type=cmult
  Register : xbsIndex_r4/Register  init=real(M3(1,5))  rst=off  en=off  dbl_ovrd=off  block_type=register
  Register1 : xbsIndex_r4/Register  init=0  rst=off  en=off  dbl_ovrd=off  block_type=register
  w_ij(n)*Gy(n)2 : xbsIndex_r4/Mult  precision=User Defined  arith_type="Signed  (2's comp)"  n_bits=nb  bin_pt=bp  quantization="Round  (unbiased: +/- Inf)"  overflow=Saturate  en=off  latency=delayMulx  dbl_ovrd=off  use_behavioral_HDL=off  opt=Speed  use_embedded=on  optimum_pipeline=off  pipeline=on  use_rpm=on  placement_style=Triangular  block_type=mult
  Wx_11(n) : Outport
  wires:
  Gx_1(n)/1 -> w_ij(n)*Gy(n)2/1
  Register/1 -> Wx_11(n)/1, Register1/1, AddSub1/1  "w_ij(n)"
  CMult2/1 -> AddSub2/1  "alpha*w_ij(n-1)"
  Register1/1 -> CMult2/1  "w_ij(n-1)"
  AddSub1/1 -> Register/1  "w_ij(n+1)"
  AddSub2/1 -> AddSub1/2
  CMult/1 -> AddSub2/2  "dw(n) = z_0(n)*e(n)*mu"
  w_ij(n)*Gy(n)2/1 -> CMult/1
  x_1(n)/1 -> w_ij(n)*Gy(n)2/2
